simulink model "ungatdm"  (R2018a)
settings: Solver=VariableStepAuto  StartTime=0.0  StopTime=8  FixedStep=0.001  MaxStep=0.01  RelTol=1e-3
libraries: dsparch4 x4, commchan3 x1, simulink x1
settings Model: Creator=ASUS  LastModifiedBy=Boss Tommy

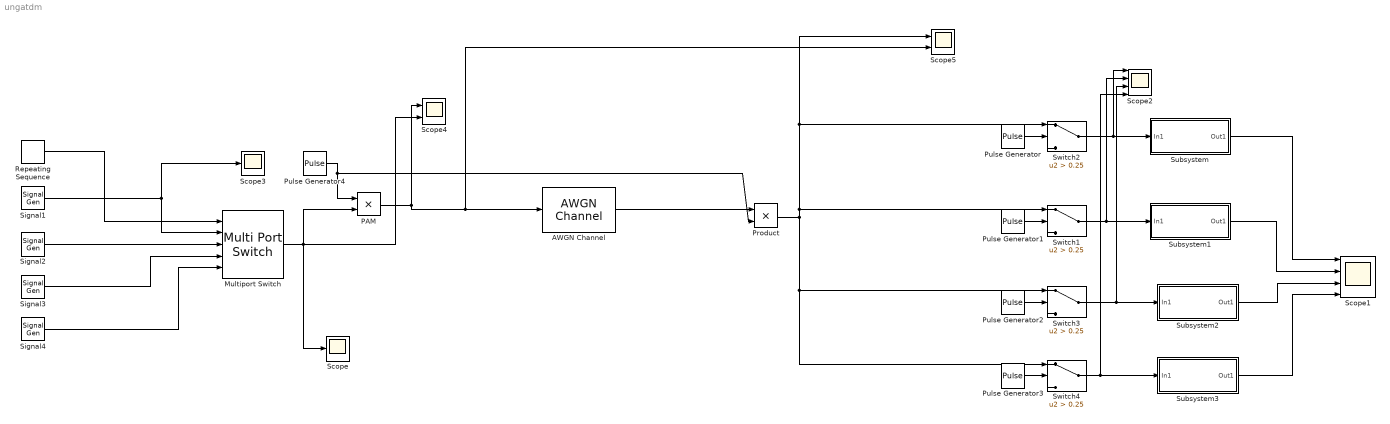
== system ungatdm ==
  AWGN Channel : commchan3/AWGN Channel  InputProcessing=Columns as channels (frame based)  seed=67  noiseMode="Signal to noise ratio  (SNR)"  EbNodB=10  EsNodB=10  SNRdB=20  bitsPerSym=1  Ps=1  Tsym=1  variance=1
  Multiport Switch : MultiPortSwitch  Inputs=4  DiagnosticForDefault=None
  PAM : Product
  Product : Product
  Pulse Generator : DiscretePulseGenerator  PulseType=Time based  Period=4  PulseWidth=24  PhaseDelay=0.05
  Pulse Generator1 : DiscretePulseGenerator  PulseType=Time based  Period=4  PulseWidth=25  PhaseDelay=1
  Pulse Generator2 : DiscretePulseGenerator  PulseType=Time based  Period=4  PulseWidth=25  PhaseDelay=2
  Pulse Generator3 : DiscretePulseGenerator  PulseType=Time based  Period=4  PulseWidth=25  PhaseDelay=3
  Pulse Generator4 : DiscretePulseGenerator  PulseType=Time based  Amplitude=1.16  Period=1/30  PulseWidth=25
  Repeating Sequence : simulink/Sources/Repeating Sequence  rep_seq_t=[1 2 3 4 5]  rep_seq_y=[1 2 3 4 5]
  Scope : Scope
  Scope1 : Scope  NumInputPorts=4
  Scope2 : Scope  NumInputPorts=4
  Scope3 : Scope
  Scope4 : Scope  NumInputPorts=2
  Scope5 : Scope  NumInputPorts=2
  Signal1 : SignalGenerator  Frequency=10
  "Signal2 " : SignalGenerator  Amplitude=2  Frequency=10
  Signal3 : SignalGenerator  Amplitude=3  Frequency=10
  "Signal4 " : SignalGenerator  Amplitude=4  Frequency=10
  Subsystem : Subsystem
  Subsystem1 : Subsystem
  Subsystem2 : Subsystem
  Subsystem3 : Subsystem
  Switch{1..4} (4 alike) : Switch  Criteria=u2 > Threshold  Threshold=0.25
  wires:
  Repeating Sequence/1 -> Multiport Switch/1
  Switch1/1 -> Subsystem1/1(In1), Scope2/2
  Switch2/1 -> Subsystem/1(In1), Scope2/1
  Multiport Switch/1 -> Scope4/2, PAM/2, Scope/1
  Pulse Generator/1 -> Switch2/2
  Pulse Generator1/1 -> Switch1/2
  Subsystem/1(Out1) -> Scope1/1
  Pulse Generator2/1 -> Switch3/2
  Pulse Generator3/1 -> Switch4/2
  Switch3/1 -> Scope2/3, Subsystem2/1(In1)
  Switch4/1 -> Scope2/4, Subsystem3/1(In1)
  Subsystem1/1(Out1) -> Scope1/2
  Subsystem2/1(Out1) -> Scope1/3
  Subsystem3/1(Out1) -> Scope1/4
  "Signal4 "/1 -> Multiport Switch/5
  Signal3/1 -> Multiport Switch/4
  "Signal2 "/1 -> Multiport Switch/3
  Signal1/1 -> Multiport Switch/2, Scope3/1
  Pulse Generator4/1 -> PAM/1, Product/2
  PAM/1 -> Scope5/2, AWGN Channel/1, Scope4/1
  Product/1 -> Scope5/1, Switch2/1, Switch1/1, Switch3/1, Switch4/1
  AWGN Channel/1 -> Product/1

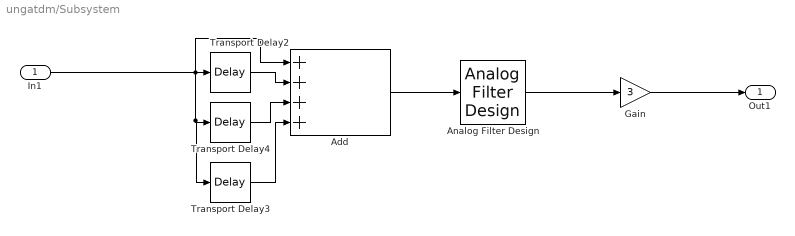
== system ungatdm/Subsystem ==
  In1 : Inport
  Add : Sum  Inputs=++++
  Analog Filter Design : dsparch4/Analog Filter Design  method=Chebyshev I  filttype=Lowpass  N=8  Wlo=2*pi*10  Whi=80  Rp=0.001  Rs=40
  Gain : Gain  Gain=3
  Transport Delay2 : TransportDelay
  Transport Delay3 : TransportDelay  DelayTime=3
  Transport Delay4 : TransportDelay  DelayTime=2
  Out1 : Outport  VectorParamsAs1DForOutWhenUnconnected=off
  wires:
  Transport Delay4/1 -> Add/3
  Transport Delay2/1 -> Add/2
  In1/1 -> Add/1, Transport Delay2/1, Transport Delay3/1, Transport Delay4/1
  Add/1 -> Analog Filter Design/1
  Transport Delay3/1 -> Add/4
  Analog Filter Design/1 -> Gain/1
  Gain/1 -> Out1/1

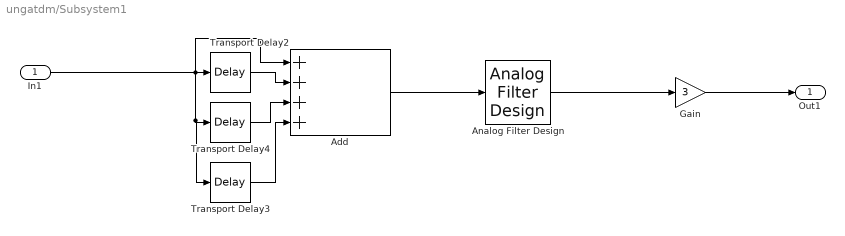
== system ungatdm/Subsystem1 ==
  In1 : Inport
  Add : Sum  Inputs=++++
  Analog Filter Design : dsparch4/Analog Filter Design  method=Chebyshev I  filttype=Lowpass  N=8  Wlo=2*pi*10  Whi=80  Rp=0.01  Rs=40
  Gain : Gain  Gain=3
  Transport Delay2 : TransportDelay
  Transport Delay3 : TransportDelay  DelayTime=3
  Transport Delay4 : TransportDelay  DelayTime=2
  Out1 : Outport  VectorParamsAs1DForOutWhenUnconnected=off
  wires:
  Transport Delay4/1 -> Add/3
  Transport Delay2/1 -> Add/2
  In1/1 -> Add/1, Transport Delay2/1, Transport Delay3/1, Transport Delay4/1
  Transport Delay3/1 -> Add/4
  Add/1 -> Analog Filter Design/1
  Analog Filter Design/1 -> Gain/1
  Gain/1 -> Out1/1

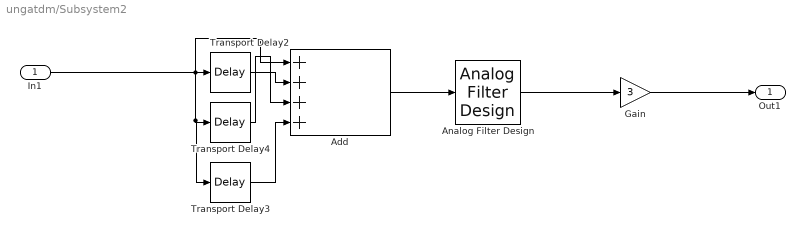
== system ungatdm/Subsystem2 ==
  In1 : Inport
  Add : Sum  Inputs=++++
  Analog Filter Design : dsparch4/Analog Filter Design  method=Chebyshev I  filttype=Lowpass  N=8  Wlo=2*pi*10  Whi=80  Rp=0.001  Rs=40
  Gain : Gain  Gain=3
  Transport Delay2 : TransportDelay
  Transport Delay3 : TransportDelay  DelayTime=3
  Transport Delay4 : TransportDelay  DelayTime=2
  Out1 : Outport
  wires:
  Transport Delay4/1 -> Add/3
  Transport Delay2/1 -> Add/2
  In1/1 -> Add/1, Transport Delay2/1, Transport Delay3/1, Transport Delay4/1
  Add/1 -> Analog Filter Design/1
  Transport Delay3/1 -> Add/4
  Analog Filter Design/1 -> Gain/1
  Gain/1 -> Out1/1

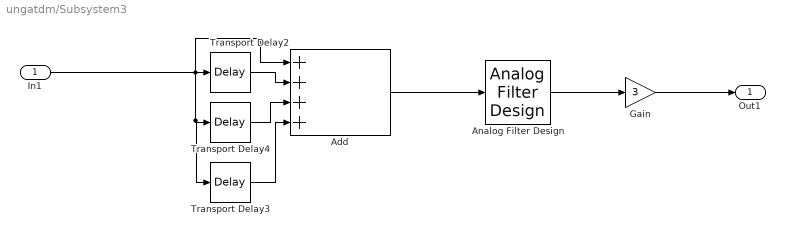
== system ungatdm/Subsystem3 ==
  In1 : Inport
  Add : Sum  Inputs=++++
  Analog Filter Design : dsparch4/Analog Filter Design  method=Chebyshev I  filttype=Lowpass  N=8  Wlo=2*pi*10  Whi=80  Rp=0.001  Rs=40
  Gain : Gain  Gain=3
  Transport Delay2 : TransportDelay
  Transport Delay3 : TransportDelay  DelayTime=3
  Transport Delay4 : TransportDelay  DelayTime=2
  Out1 : Outport  VectorParamsAs1DForOutWhenUnconnected=off
  wires:
  Transport Delay4/1 -> Add/3
  Transport Delay2/1 -> Add/2
  In1/1 -> Add/1, Transport Delay2/1, Transport Delay3/1, Transport Delay4/1
  Transport Delay3/1 -> Add/4
  Add/1 -> Analog Filter Design/1
  Analog Filter Design/1 -> Gain/1
  Gain/1 -> Out1/1
